simulink model "SwimmingPoolSimulationModel"  (R2018b)
settings: Solver=VariableStepAuto  StartTime=0.0  StopTime=4320000  MaxStep=100  RelTol=1e-3  AbsTol=1e-3  EnableMultiTasking=on
values from neighbouring files (symbols this model uses):
  A_tank = 2*w*h + 2*l*h + l*w    (= 68.7)    [SwimmingPoolSimulation.m]
  A_water = l*w    (= 32.4)    [SwimmingPoolSimulation.m]
  c_water = 4184    [SwimmingPoolSimulation.m]
  Dh = 2*r    (= 0.1)    [SwimmingPoolSimulation.m]
  h = 1.5    [SwimmingPoolSimulation.m]
  H_length = 0.5    [SwimmingPoolSimulation.m]
  l = 8.1    [SwimmingPoolSimulation.m]
  m_ev = (109.6 + 3.9) / 50    (= 2.27)    [SwimmingPoolSimulation.m]
  P_air_ground = pi/4    (= 0.785398163397)    [SwimmingPoolSimulation.m]
  P_Smax = absorption*P_Sperp    [SwimmingPoolSimulation.m]
  PA = r^2 * pi    (= 0.00785398163397)    [SwimmingPoolSimulation.m]
  q_water = 2257e3    (= 2257000)    [SwimmingPoolSimulation.m]
  Rth_G = 2    [SwimmingPoolSimulation.m]
  T_Amax = 19    [SwimmingPoolSimulation.m]
  T_Amin = 8    [SwimmingPoolSimulation.m]
  T_Gmax = (T_Amax + T_Amin)/2 + 1    (= 14.5)    [SwimmingPoolSimulation.m]
  T_Gmin = (T_Amax + T_Amin)/2 - 1    (= 12.5)    [SwimmingPoolSimulation.m]
  w = 4    [SwimmingPoolSimulation.m]
libraries: fl_lib x18, nesl_utility x8, SimscapeFluids_lib x2
settings Model: Creator=me  LastModifiedBy=nicoc
settings SolverCC: AutoScaleAbsTol=off
settings DataIOCC: LimitDataPoints=on  MaxDataPoints=10000
settings OptimizationCC: LifeSpan=inf
settings DebuggingCC: AllowSymbolicDim=off  LibraryContextMissingDiagnostic=none  SFUnexpectedBacktrackingDiag=warning  SFNoUnconditionalDefaultTransitionDiag=warning  SFExecutionAtInitializationDiag=none
settings SFSimCC: SimUseLocalCustomCode=off
settings RTWCC: RTWUseLocalCustomCode=off
settings CodeAppCC: StateflowObjectComments=on
settings GRTTargetCC: TargetLangStandard=C89/C90 (ANSI)  GeneratePreprocessorConditionals=Disable all
settings ConfigComp: CovMetricSettings=dw  CovHtmlReporting=on  CovSaveCumulativeToWorkspaceVar=on  CovSaveSingleToWorkspaceVar=on  CovExternalEMLEnable=off  CovSFcnEnable=off
settings SimscapeCC: SimscapeLogType=all  SimscapeLogLimitData=off  SimscapeLogDataHistory=10000

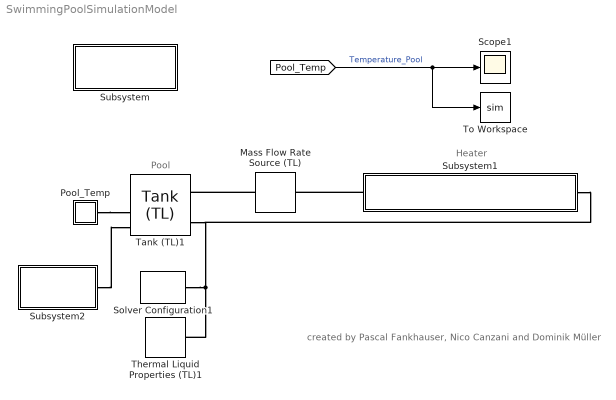
== system SwimmingPoolSimulationModel ==
  note: Pool
  note: created by Pascal Fankhauser, Nico Canzani and Dominik Müller
  note: Heater
  Mass Flow Rate Source (TL) : fl_lib/Thermal Liquid/Sources/Mass Flow Rate Source (TL)  commanded_mass_flow=MFR kg/s  area=PA m^2  length=0.1 m  mdot_A_specify=off  mdot_A_priority=None  mdot_A=1 kg/s  mdot_A_nominal_specify=off  mdot_A_nominal_unit=kg/s  mdot_A_nominal_value=1
      settings: SourceProductName=Simscape  SourceProductBaseCode=SS
  Pool_Temp : Subsystem  Description=Simscape Probe  InitFcn=|
      | unit=get_param([gcb '/PS-S'],'Unit');                                              
      | set_param(gcb, 'AttributesFormatString', strcat('[', unit,']'));
      mask help: Simscape Probe
      settings: AttributesFormatString=[1]
      settings: CopyFcn=|
      | if strcmp(get_param(gcb, 'LinkStatus'),'implicit') == 0;
      | set_param(gcb,'LinkStatus','inactive');
      | set_param(gcb,'LinkStatus','none');
      | end
      | set_param([gcb '/Goto'],'GotoTag', [get(gcbh,'name')]);
      | set_param([gcb '/From'],'GotoTag', [get(gcbh,'name')]);
      | h = get_param([gcb, '/PS-S'], 'PortHandles');
      | set(h.Outport(1), 'SignalNameFromLabel', [get(gcbh,'name')])
      | clear h;
      settings: NameChangeFcn=|
      | set_param([gcb '/Goto'],'GotoTag', [get(gcbh,'name')]);
      | set_param([gcb '/From'],'GotoTag', [get(gcbh,'name')]);
      | h = get_param([gcb, '/PS-S'], 'PortHandles');
      | set(h.Outport(1), 'SignalNameFromLabel', [get(gcbh,'name')])
      | clear h;
      settings: OpenFcn=|
      | if exist('logsout', 'var')
      |   vname = get(gcbh,'name');
      |   fHandle = findall(0,'Tag',vname);
      |   if isempty(fHandle)
      |   figure('Tag',vname);
      |   end;
      |   figure(findobj('Tag',vname));
      |   plot(logsout.getElement([gcb, '/PS-S'], '-blockpath').Values)
      |   title(get(gcbh,'name'));
      |   ylabel(['Physical Signal (' get_param([gcb '/PS-S'],'Unit') ')'] );
      | end
      mask Display: disp('PS');
  Scope1 : Scope
  Solver Configuration1 : nesl_utility/Solver Configuration  PhysicalDomain=network_engine_domain  SubClassName=solver  LeftPortType=input  RightPortType=generic  Tones=[]  Harmonics=[]  SimulateNoise=off  Profile=off  UseLocalSampling=off  EnableSwitchedLinearOptims=on  FrequencyDomain=off  UseCCode=off  RelTol=0.001  AbsTol=1e-06  MinStep=1e-09  ToWorkspace=off  RevertToSquareIcSolve=off  NumHomotopyIterations=100  PhasorMode=off  PhasorModeNumHarmonics=1  DoDC=off  ResidualTolerance=1e-09  UseLocalSolver=off  LocalSolverChoice=NE_BACKWARD_EULER_ADVANCER  LocalSolverSampleTime=0.001  DoFixedCost=off  MaxNonlinIter=3  MaxModeIter=2  LinearAlgebra=auto  EquationFormulation=NE_TIME_EF  DelaysMemoryBudget=1024  AutomaticFiltering=on  FilteringTimeConstant=0.001  PartitionStorageMethod=AS_NEEDED  PartitionMemoryBudget=1024
  Subsystem : Subsystem
      settings: OpenFcn=open_system('simscape')
      mask Display: disp(sprintf('Open Simscape\nLibrary'));
  Subsystem1 : Subsystem
  Subsystem2 : Subsystem
  Tank (TL)1 : SimscapeFluids_lib/Thermal Liquid/Tanks & Accumulators/Tank (TL)  pressure_spec=1  tank_pressure=0.101325 MPa  max_capacity=1.1*l*w*h m^3  volume_spec=1  tank_area=l*w m^2  level_TLU=[0, 3, 5] m  volume_TLU=[0, 4, 6] m^3  inlet_height=[0.1 0.1] m  inlet_area=0.01 m^2  g=9.81 m/s^2  level_specify=on  level_priority=None  level=h m  level_nominal_specify=off  level_nominal_unit=m  level_nominal_value=1  volume_specify=on  volume_priority=High  volume=l*w*h m^3  volume_nominal_specify=off  volume_nominal_unit=m^3  volume_nominal_value=1  mass_specify=on  mass_priority=None  mass=1000*l*w*h kg  mass_nominal_specify=off  mass_nominal_unit=kg  mass_nominal_value=1  T_tank_specify=on  T_tank_priority=High  T_tank=283.15 K  T_tank_nominal_specify=off  T_tank_nominal_unit=K  T_tank_nominal_value=1  inlet_heights_AB=[1.4, 0.2] m  inlet_areas_AB=[PA, PA] m^2  inlet_heights_ABC=[.1, .05, 0] m  inlet_areas_ABC=[.01, .01, .01] m^2
      settings: SourceProductName=Simscape Fluids  SourceProductBaseCode=SH
  Thermal Liquid Properties (TL)1 : SimscapeFluids_lib/Thermal Liquid/Utilities/Thermal Liquid Properties (TL)  fluid_list=1  concentration_param_EG=1  concentration_param_PG=1  c_mass_SW=3.5e-3  c_mass_EG=0.1  c_mass_PG=0.1  c_mass_GL=0.1  c_vol_EG=0.1  c_vol_PG=0.1  beta_const_EG=2.1791 GPa  beta_const_PG=2.1791 GPa  beta_const_GL=2.1791 GPa  p_min_EG=0.01 MPa  p_min_PG=0.01 MPa  p_min_GL=0.01 MPa  p_max_EG=50 MPa  p_max_PG=50 MPa  p_max_GL=50 MPa  p_atm=101.325 kPa
      settings: SourceProductName=Simscape Fluids  SourceProductBaseCode=SH
  To Workspace : ToWorkspace  VariableName=sim  SaveFormat=Timeseries  SampleTime=-1
  wires:
  [Pool_Temp] -> To Workspace/1, Scope1/1  "Temperature_Pool"
  connections:
  Mass Flow Rate Source (TL)/LConn1 -- Tank (TL)1/LConn1
  Pool_Temp/LConn1 -- Tank (TL)1/RConn3
  Subsystem2/LConn1 -- Tank (TL)1/RConn4
  Subsystem1/LConn1 -- Mass Flow Rate Source (TL)/RConn1
  Solver Configuration1/RConn1 -- Subsystem1/RConn1 -- Tank (TL)1/LConn2 -- Thermal Liquid Properties (TL)1/RConn1

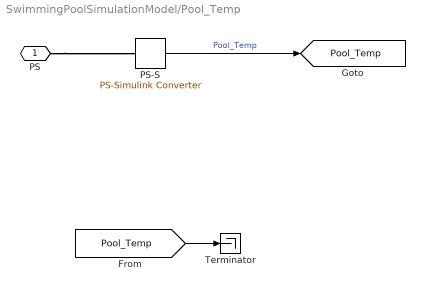
== system SwimmingPoolSimulationModel/Pool_Temp ==
  PS-S : nesl_utility/PS-Simulink Converter  PhysicalDomain=network_engine_domain  SubClassName=ps_output  LeftPortType=input  RightPortType=output  PseudoPeriodic=off  Frequencies=[]  Unit=1  AffineConversion=off
  Terminator : Terminator
  PS : PMIOPort  Side=Left
  tag scope: Pool_Temp=global
  wires:
  [Pool_Temp] -> Terminator/1
  PS-S/1 -> [Pool_Temp]  "Pool_Temp"
  connections:
  PS/RConn1 -- PS-S/LConn1

== system SwimmingPoolSimulationModel/Subsystem ==

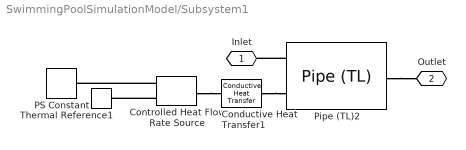
== system SwimmingPoolSimulationModel/Subsystem1 ==
  Conductive Heat Transfer1 : fl_lib/Thermal/Thermal Elements/Conductive Heat Transfer  area=Dh*pi*H_length m^2  thickness=0.01 m  th_cond=401 W/(m*K)  T_specify=off  T_priority=None  T=0 K  T_nominal_specify=off  T_nominal_unit=K  T_nominal_value=1  Q_specify=off  Q_priority=None  Q=0 W  Q_nominal_specify=off  Q_nominal_unit=W  Q_nominal_value=1
      settings: SourceProductName=Simscape
  Controlled Heat Flow Rate Source : fl_lib/Thermal/Thermal Sources/Controlled Heat Flow Rate Source
      settings: SourceProductName=Simscape
  PS Constant : fl_lib/Physical Signals/Sources/PS Constant  constant=P_Heater
  Pipe (TL)2 : fl_lib/Thermal Liquid/Elements/Pipe (TL)  dynamic_compressibility=1  inertia=0  length=H_length m  area=PA m^2  Dh=Dh m  length_add=1 m  roughness=15e-6 m  Re_lam=2000  Re_tur=4000  shape_factor=64  Nu_lam=3.66  p0=0.101325 MPa  T0=283.15 K  mdot0=0 kg/s
      settings: SourceProductName=Simscape  SourceProductBaseCode=SS
  Thermal Reference1 : fl_lib/Thermal/Thermal Elements/Thermal Reference
  Inlet : PMIOPort  Side=Left
  Outlet : PMIOPort  Port=2  Side=Right
  connections:
  Controlled Heat Flow Rate Source/LConn1 -- Conductive Heat Transfer1/LConn1
  Pipe (TL)2/RConn1 -- Outlet/RConn1
  Controlled Heat Flow Rate Source/RConn2 -- Thermal Reference1/LConn1
  Pipe (TL)2/LConn1 -- Inlet/RConn1
  Conductive Heat Transfer1/RConn1 -- Pipe (TL)2/LConn2
  Controlled Heat Flow Rate Source/RConn1 -- PS Constant/RConn1

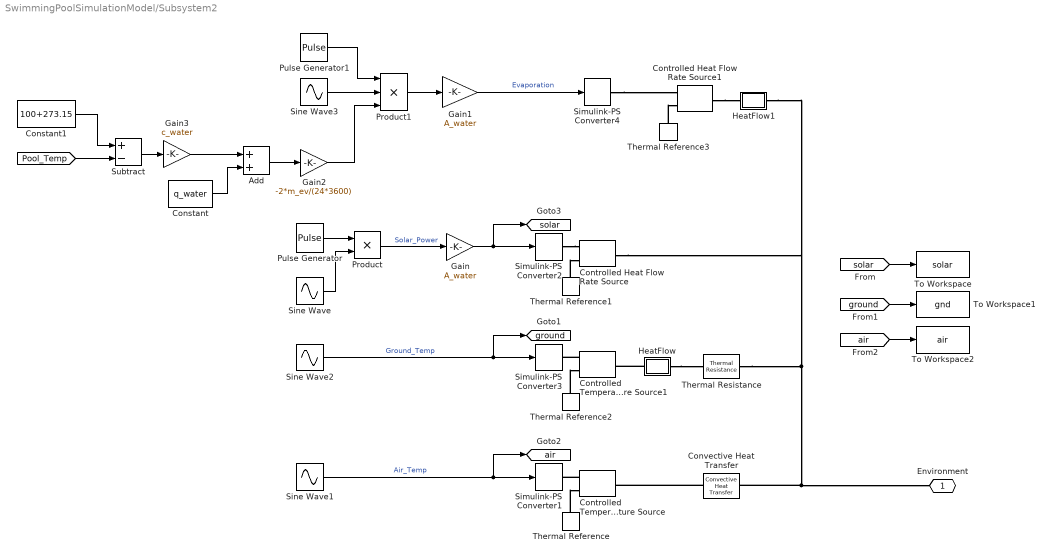
== system SwimmingPoolSimulationModel/Subsystem2 ==
  Add : Sum
  Constant : Constant  Value=q_water
  Constant1 : Constant  Value=100+273.15
  Controlled Temperature Source : fl_lib/Thermal/Thermal Sources/Controlled Temperature Source
      settings: SourceProductName=Simscape
  Controlled Temperature Source1 : fl_lib/Thermal/Thermal Sources/Controlled Temperature Source
      settings: SourceProductName=Simscape
  Controlled Heat Flow Rate Source : fl_lib/Thermal/Thermal Sources/Controlled Heat Flow Rate Source
      settings: SourceProductName=Simscape
  Controlled Heat Flow Rate Source1 : fl_lib/Thermal/Thermal Sources/Controlled Heat Flow Rate Source
      settings: SourceProductName=Simscape
  Convective Heat Transfer : fl_lib/Thermal/Thermal Elements/Convective Heat Transfer  area=l*w m^2  heat_tr_coeff=h_pool_air W/(m^2 * K)  T_specify=off  T_priority=None  T=0 K  T_nominal_specify=off  T_nominal_unit=K  T_nominal_value=1  Q_specify=off  Q_priority=None  Q=0 W  Q_nominal_specify=off  Q_nominal_unit=W  Q_nominal_value=1
  Gain : Gain  Gain=A_water
  Gain1 : Gain  Gain=A_water
  Gain2 : Gain  Gain=-2*m_ev/(24*3600)
  Gain3 : Gain  Gain=c_water
  HeatFlow : Subsystem  Description=Simscape Probe  InitFcn=|
      | unit=get_param([gcb '/PS-S'],'Unit');                                              
      | set_param(gcb, 'AttributesFormatString', strcat('[', unit,']'));
      mask help: Simscape Probe
      settings: AttributesFormatString=[J/s]
      settings: CopyFcn=|
      | if strcmp(get_param(gcb, 'LinkStatus'),'implicit') == 0;
      | set_param(gcb,'LinkStatus','inactive');
      | set_param(gcb,'LinkStatus','none');
      | end
      | set_param([gcb '/Goto'],'GotoTag', [get(gcbh,'name')]);
      | set_param([gcb '/From'],'GotoTag', [get(gcbh,'name')]);
      | h = get_param([gcb, '/PS-S'], 'PortHandles');
      | set(h.Outport(1), 'SignalNameFromLabel', [get(gcbh,'name')])
      | clear h;
      settings: NameChangeFcn=|
      | set_param([gcb '/Goto'],'GotoTag', [get(gcbh,'name')]);
      | set_param([gcb '/From'],'GotoTag', [get(gcbh,'name')]);
      | h = get_param([gcb, '/PS-S'], 'PortHandles');
      | set(h.Outport(1), 'SignalNameFromLabel', [get(gcbh,'name')])
      | clear h;
      settings: OpenFcn=|
      | if exist('logsout', 'var')
      |   vname = get(gcbh,'name');
      |   fHandle = findall(0,'Tag',vname);
      |   if isempty(fHandle)
      |   figure('Tag',vname);
      |   end;
      |   figure(findobj('Tag',vname));
      |   plot(logsout.getElement([gcb, '/PS-S'], '-blockpath').Values)
      |   title(get(gcbh,'name'));
      |   ylabel(['Heat Flow (' get_param([gcb '/PS-S'],'Unit') ')'] );
      | end
      mask Display:
      | patch([0.5 1 0.5], [0.25 .5 0.75],[0.7 0.7 0.7])
      | plot([0,0.5],[0.5,0.5]);
  HeatFlow1 : Subsystem  Description=Simscape Probe  InitFcn=|
      | unit=get_param([gcb '/PS-S'],'Unit');                                              
      | set_param(gcb, 'AttributesFormatString', strcat('[', unit,']'));
      mask help: Simscape Probe
      settings: AttributesFormatString=[J/s]
      settings: CopyFcn=|
      | if strcmp(get_param(gcb, 'LinkStatus'),'implicit') == 0;
      | set_param(gcb,'LinkStatus','inactive');
      | set_param(gcb,'LinkStatus','none');
      | end
      | set_param([gcb '/Goto'],'GotoTag', [get(gcbh,'name')]);
      | set_param([gcb '/From'],'GotoTag', [get(gcbh,'name')]);
      | h = get_param([gcb, '/PS-S'], 'PortHandles');
      | set(h.Outport(1), 'SignalNameFromLabel', [get(gcbh,'name')])
      | clear h;
      settings: NameChangeFcn=|
      | set_param([gcb '/Goto'],'GotoTag', [get(gcbh,'name')]);
      | set_param([gcb '/From'],'GotoTag', [get(gcbh,'name')]);
      | h = get_param([gcb, '/PS-S'], 'PortHandles');
      | set(h.Outport(1), 'SignalNameFromLabel', [get(gcbh,'name')])
      | clear h;
      settings: OpenFcn=|
      | if exist('logsout', 'var')
      |   vname = get(gcbh,'name');
      |   fHandle = findall(0,'Tag',vname);
      |   if isempty(fHandle)
      |   figure('Tag',vname);
      |   end;
      |   figure(findobj('Tag',vname));
      |   plot(logsout.getElement([gcb, '/PS-S'], '-blockpath').Values)
      |   title(get(gcbh,'name'));
      |   ylabel(['Heat Flow (' get_param([gcb '/PS-S'],'Unit') ')'] );
      | end
      mask Display:
      | patch([0.5 1 0.5], [0.25 .5 0.75],[0.7 0.7 0.7])
      | plot([0,0.5],[0.5,0.5]);
  Product : Product
  Product1 : Product  Inputs=3
  Pulse Generator : DiscretePulseGenerator  PulseType=Time based  Period=24*3600  PulseWidth=50
  Pulse Generator1 : DiscretePulseGenerator  PulseType=Time based  Period=60*60*24  PulseWidth=50
  Simulink-PS Converter1 : nesl_utility/Simulink-PS Converter  PhysicalDomain=network_engine_domain  SubClassName=ps_input  LeftPortType=input  RightPortType=output  PseudoPeriodic=off  Frequencies=[]  NoiseDistribution=none  NoiseParameters=[]  Unit=degC  AffineConversion=on  FilteringAndDerivatives=zero  SimscapeFilterOrder=1  InputFilterTimeConstant=.001  UdotUserProvided=0
  Simulink-PS Converter2 : nesl_utility/Simulink-PS Converter  PhysicalDomain=network_engine_domain  SubClassName=ps_input  LeftPortType=input  RightPortType=output  PseudoPeriodic=off  Frequencies=[]  NoiseDistribution=none  NoiseParameters=[]  Unit=J/s  AffineConversion=on  FilteringAndDerivatives=zero  SimscapeFilterOrder=1  InputFilterTimeConstant=.001  UdotUserProvided=0
  Simulink-PS Converter3 : nesl_utility/Simulink-PS Converter  PhysicalDomain=network_engine_domain  SubClassName=ps_input  LeftPortType=input  RightPortType=output  PseudoPeriodic=off  Frequencies=[]  NoiseDistribution=none  NoiseParameters=[]  Unit=degC  AffineConversion=on  FilteringAndDerivatives=zero  SimscapeFilterOrder=1  InputFilterTimeConstant=.001  UdotUserProvided=0
  Simulink-PS Converter4 : nesl_utility/Simulink-PS Converter  PhysicalDomain=network_engine_domain  SubClassName=ps_input  LeftPortType=input  RightPortType=output  PseudoPeriodic=off  Frequencies=[]  NoiseDistribution=none  NoiseParameters=[]  Unit=J/s  AffineConversion=on  FilteringAndDerivatives=zero  SimscapeFilterOrder=1  InputFilterTimeConstant=.001  UdotUserProvided=0
  Sine Wave : Sin  Amplitude=P_Smax/2  Bias=P_Smax/2  Frequency=2*pi/(12*3600)  Phase=-pi/2  SampleTime=0
  Sine Wave1 : Sin  Amplitude=(T_Amax - T_Amin)/2  Bias=(T_Amax + T_Amin)/2  Frequency=2*pi/(24*3600)  Phase=-pi/2  SampleTime=0
  Sine Wave2 : Sin  Amplitude=(T_Gmax - T_Gmin)/2  Bias=(T_Gmax + T_Gmin)/2  Frequency=2*pi/(24*3600)  Phase=-pi/2 - P_air_ground  SampleTime=0
  Sine Wave3 : Sin  Bias=1  Frequency=2*pi/(60*60*12)  Phase=-pi/2  SampleTime=0
  Subtract : Sum  Inputs=+-
  Thermal Reference{,1..3} (4 alike) : fl_lib/Thermal/Thermal Elements/Thermal Reference
  Thermal Resistance : fl_lib/Thermal/Thermal Elements/Thermal Resistance  resistance=Rth_G/A_tank K/W  T_specify=off  T_priority=None  T=0 K  T_nominal_specify=off  T_nominal_unit=K  T_nominal_value=1  Q_specify=off  Q_priority=None  Q=0 W  Q_nominal_specify=off  Q_nominal_unit=W  Q_nominal_value=1
      settings: SourceProductName=Simscape  SourceProductBaseCode=SS
  To Workspace : ToWorkspace  VariableName=solar  SaveFormat=Timeseries  SampleTime=-1
  To Workspace1 : ToWorkspace  VariableName=gnd  SaveFormat=Timeseries  SampleTime=-1
  To Workspace2 : ToWorkspace  VariableName=air  SaveFormat=Timeseries  SampleTime=-1
  Environment : PMIOPort  Side=Left
  tag scope: air=global, ground=global, solar=global
  wires:
  Sine Wave1/1 -> Simulink-PS Converter1/1, [air]  "Air_Temp"
  Sine Wave2/1 -> [ground], Simulink-PS Converter3/1  "Ground_Temp"
  Pulse Generator/1 -> Product/1
  Sine Wave/1 -> Product/2
  Product/1 -> Gain/1  "Solar_Power"
  Gain/1 -> Simulink-PS Converter2/1, [solar]
  [solar] -> To Workspace/1
  [ground] -> To Workspace1/1
  [air] -> To Workspace2/1
  Pulse Generator1/1 -> Product1/1
  Sine Wave3/1 -> Product1/2
  Product1/1 -> Gain1/1
  Gain1/1 -> Simulink-PS Converter4/1  "Evaporation"
  Add/1 -> Gain2/1
  Constant/1 -> Add/2
  Constant1/1 -> Subtract/1
  [Pool_Temp] -> Subtract/2
  Subtract/1 -> Gain3/1
  Gain3/1 -> Add/1
  Gain2/1 -> Product1/3
  connections:
  Thermal Resistance/RConn1 -- HeatFlow1/RConn1 -- Controlled Heat Flow Rate Source/LConn1 -- Environment/RConn1 -- Convective Heat Transfer/LConn1
  Thermal Reference2/LConn1 -- Controlled Temperature Source1/RConn2
  Convective Heat Transfer/RConn1 -- Controlled Temperature Source/LConn1
  Thermal Reference1/LConn1 -- Controlled Heat Flow Rate Source/RConn2
  Controlled Temperature Source/RConn1 -- Simulink-PS Converter1/RConn1
  Simulink-PS Converter2/RConn1 -- Controlled Heat Flow Rate Source/RConn1
  Controlled Temperature Source1/RConn1 -- Simulink-PS Converter3/RConn1
  Thermal Reference/LConn1 -- Controlled Temperature Source/RConn2
  Simulink-PS Converter4/RConn1 -- Controlled Heat Flow Rate Source1/RConn1
  Thermal Reference3/LConn1 -- Controlled Heat Flow Rate Source1/RConn2
  HeatFlow/LConn1 -- Controlled Temperature Source1/LConn1
  HeatFlow/RConn1 -- Thermal Resistance/LConn1
  Controlled Heat Flow Rate Source1/LConn1 -- HeatFlow1/LConn1

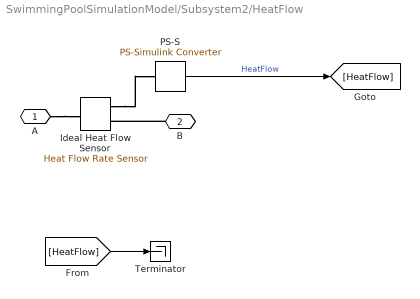
== system SwimmingPoolSimulationModel/Subsystem2/HeatFlow ==
  Ideal Heat Flow Sensor : fl_lib/Thermal/Thermal Sensors/Heat Flow Rate Sensor
      settings: SourceProductName=Simscape  SourceProductBaseCode=SS
  PS-S : nesl_utility/PS-Simulink Converter  PhysicalDomain=network_engine_domain  SubClassName=ps_output  LeftPortType=input  RightPortType=output  PseudoPeriodic=off  Frequencies=[]  Unit=J/s  AffineConversion=off
  Terminator : Terminator
  A : PMIOPort  Side=Left
  B : PMIOPort  Port=2  Side=Right
  wires:
  [HeatFlow] -> Terminator/1
  PS-S/1 -> [HeatFlow]  "HeatFlow"
  connections:
  B/RConn1 -- Ideal Heat Flow Sensor/RConn2
  Ideal Heat Flow Sensor/RConn1 -- PS-S/LConn1
  A/RConn1 -- Ideal Heat Flow Sensor/LConn1

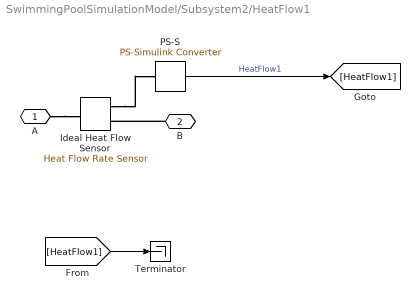
== system SwimmingPoolSimulationModel/Subsystem2/HeatFlow1 ==
  Ideal Heat Flow Sensor : fl_lib/Thermal/Thermal Sensors/Heat Flow Rate Sensor
      settings: SourceProductName=Simscape  SourceProductBaseCode=SS
  PS-S : nesl_utility/PS-Simulink Converter  PhysicalDomain=network_engine_domain  SubClassName=ps_output  LeftPortType=input  RightPortType=output  PseudoPeriodic=off  Frequencies=[]  Unit=J/s  AffineConversion=off
  Terminator : Terminator
  A : PMIOPort  Side=Left
  B : PMIOPort  Port=2  Side=Right
  wires:
  [HeatFlow1] -> Terminator/1
  PS-S/1 -> [HeatFlow1]  "HeatFlow1"
  connections:
  B/RConn1 -- Ideal Heat Flow Sensor/RConn2
  Ideal Heat Flow Sensor/RConn1 -- PS-S/LConn1
  A/RConn1 -- Ideal Heat Flow Sensor/LConn1
